simulink model "ASML_Simulate_KFilter"  (R2022a)
settings: Solver=FixedStepAuto  StartTime=0.0  StopTime=1  FixedStep=Ts  RelTol=1e-3
model workspace (MAT data in the model file):
  enab = 1
  eol = 6
  euvTarget = Simulink.Parameter
  euvTarget.Value = 4.4
  euvTarget.DataType = 'auto'
  euvTarget.Complexity = 'real'
  euvTarget.Dimensions = [1 1]
values from neighbouring files (symbols this model uses):
  euvTarget = 5    [modelParams.mat]
  HitDelayMode = 'zeroShot'    [modelParams.mat]    (also in variantParams.mat)
  SenseDelayMode = 'twoShot'    [modelParams.mat]    (also in variantParams.mat)
  Ts = 20e-6    (= 2e-05)    [computeDose1Burst.m]    (also in computeDose1Burst_filtered.m; modelParams.mat)
undefined symbols (not defined in the file or in its folder): Discrete, Time
libraries: ctrlSharedLib x1, simulink x1
settings Model: Creator=rjacques  LastModifiedBy=maxcr
settings SolverCC: AlgebraicLoopSolver=TrustRegion
settings DataIOCC: ExternalInput=extInput_SimulateEuvControl  DSMLogging=off  SaveTime=off  ReturnWorkspaceOutputs=off
settings OptimizationCC: EfficientMapNaN2IntZero=off
settings DebuggingCC: AlgebraicLoopMsg=none  UnconnectedInputMsg=warning  UnconnectedOutputMsg=warning  UnconnectedLineMsg=warning  SFMachineParentedDataDiag=warning  ArithmeticOperatorsInVariantConditions=warning
settings HardwareCC: TargetBitPerPointer=64  TargetBitPerSizeT=64  TargetBitPerPtrDiffT=64  TargetLongLongMode=on  TargetIntDivRoundTo=Zero  TargetEndianess=LittleEndian  TargetWordSize=64  TargetHWDeviceType=MATLAB Host  ProdEqTarget=off
settings SFSimCC: SimUseLocalCustomCode=off  CustomCodeUndefinedFunction=UseInterfaceOnly
settings RTWCC: SystemTargetFile=accel.tlc  TemplateMakefile=accel_default_tmf  RTWVerbose=off  DLArmComputeVersion=19.05
settings CodeAppCC: MaxIdLength=128
settings STFCustomTargetCC: ConcurrentExecutionCompliant=on  MATLABClassNameForMDSCustomization=Simulink.SoftwareTarget.TargetSpecificTriggerConfigurationBase  SystemTargetFile=accel.tlc

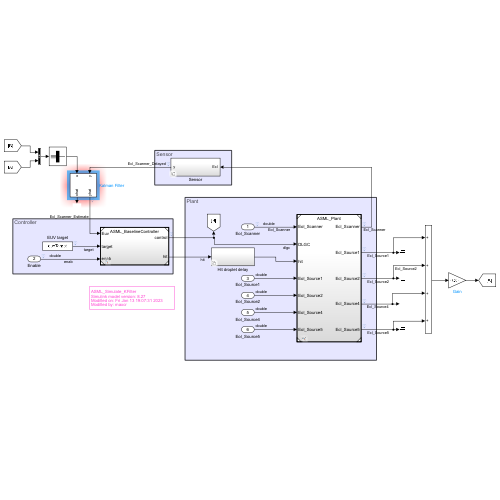
[thumbnail: Simulink's stored preview of the top-level diagram]
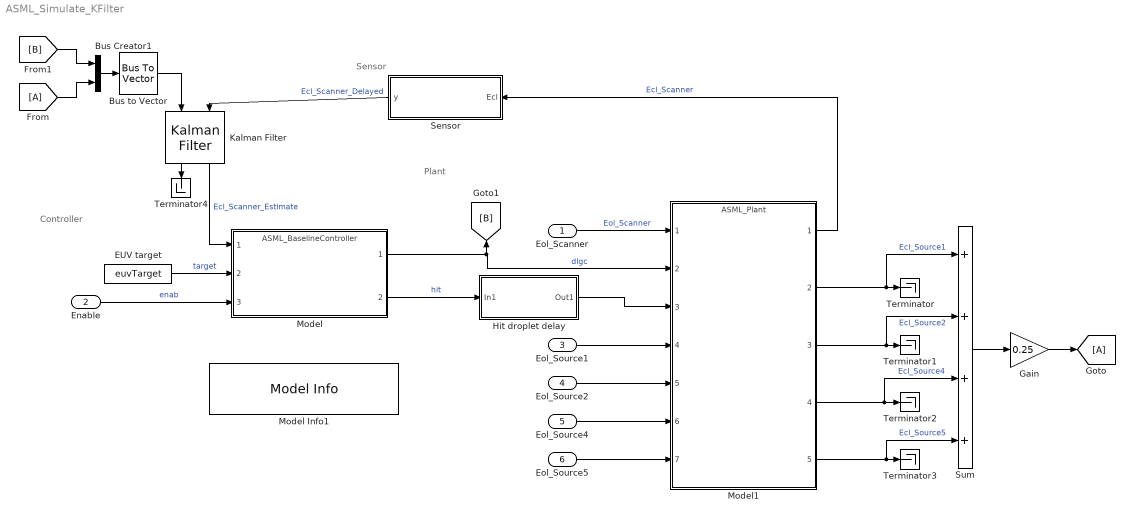
== system ASML_Simulate_KFilter ==
  note: Sensor
  note: Controller
  note: Plant
  Eol_Scanner : Inport  OutDataTypeStr=double  SampleTime=Ts
  Enable : Inport  Port=2  OutDataTypeStr=double  SampleTime=Ts
  Eol_Source1 : Inport  Port=3  OutDataTypeStr=double  SampleTime=Ts
  Eol_Source2 : Inport  Port=4  OutDataTypeStr=double  SampleTime=Ts
  Eol_Source4 : Inport  Port=5  OutDataTypeStr=double  SampleTime=Ts
  Eol_Source5 : Inport  Port=6  OutDataTypeStr=double  SampleTime=Ts
  Bus Creator1 : BusCreator  Inputs=2
  Bus to Vector : BusToVector
  EUV target : Constant  Value=euvTarget  OutDataTypeStr=double
  From : From
  Gain : Gain  Gain=0.25
  Goto : Goto
  Hit droplet delay : Subsystem  Variant=on
  Kalman Filter : ctrlSharedLib/Kalman Filter  TimeDomain=Discrete-Time  UseCurrentEstimator=off  ModelSource=LTI State-Space Variable  ModelSourceVariable=sys  A=0.95  B=1  C=1  D=0  NumberOfStates=1  NumberOfInputs=1  NumberOfOutputs=1  InitialEstimateSource=Dialog  X0=0  P0=10  UseK=off  UseGH=off  NumberOfProcessNoiseInputs=1  G=1  TimeInvariantG=on  H=0  TimeInvariantH=on  Q=0.05  TimeInvariantQ=on  R=1  TimeInvariantR=on  N=0  TimeInvariantN=on  AddInputPort=on  AddEnablePort=off  OutputEstimatedY=on  OutputP=off  Ts=-1
  Model : ModelReference  ModelNameDialog=ASML_BaselineController.slx  SimulationMode=Normal  ModelReferenceVersion=8.0
  Model Info1 : simulink/Model-Wide Utilities/Model Info  Frame=on  DisplayStringWithTags=|  HorizontalTextAlignment=Left  LeftAlignmentValue=0.02
      | %<ModelName>
      | Simulink model version: %<ModelVersion>
      | Modified on: %<LastModificationDate>
      | Modified by: %<ModifiedBy>
  Model1 : ModelReference  ModelNameDialog=ASML_Plant.slx  SimulationMode=Normal  ModelReferenceVersion=8.20
  Sensor : Subsystem  Variant=on  VariantControl=Variant1
  Sum : Sum  Inputs=++++
  Terminator{,1..4} (5 alike) : Terminator
  wires:
  Model/1 -> Model1/2, [B]  "dlgc"
  Eol_Scanner/1 -> Model1/1  "Eol_Scanner"
  EUV target/1 -> Model/2  "target"
  Model1/1 -> Sensor/1("Ecl ")  "Ecl_Scanner"
  Model/2 -> Hit droplet delay/1(In1)  "hit"
  Hit droplet delay/1(Out1) -> Model1/3
  Sensor/1(" y") -> Kalman Filter/2  "Ecl_Scanner_Delayed"
  Enable/1 -> Model/3  "enab"
  Eol_Source1/1 -> Model1/4
  Eol_Source2/1 -> Model1/5
  Eol_Source4/1 -> Model1/6
  Eol_Source5/1 -> Model1/7
  Model1/3 -> Sum/2, Terminator1/1  "Ecl_Source2"
  Model1/4 -> Sum/3, Terminator2/1  "Ecl_Source4"
  Model1/5 -> Sum/4, Terminator3/1  "Ecl_Source5"
  Model1/2 -> Sum/1, Terminator/1  "Ecl_Source1"
  Kalman Filter/2 -> Model/1  "Ecl_Scanner_Estimate"
  Bus Creator1/1 -> Bus to Vector/1
  Bus to Vector/1 -> Kalman Filter/1
  From/1 -> Bus Creator1/2
  [B] -> Bus Creator1/1
  Kalman Filter/1 -> Terminator4/1
  Sum/1 -> Gain/1
  Gain/1 -> Goto/1

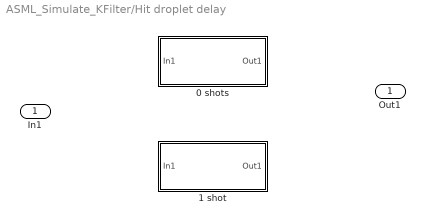
== system ASML_Simulate_KFilter/Hit droplet delay ==
  In1 : Inport
  0 shots : Subsystem  VariantControl=strcmp(HitDelayMode,'zeroShot')
  1 shot : Subsystem  VariantControl=strcmp(HitDelayMode,'oneShot')
  Out1 : Outport  VectorParamsAs1DForOutWhenUnconnected=off

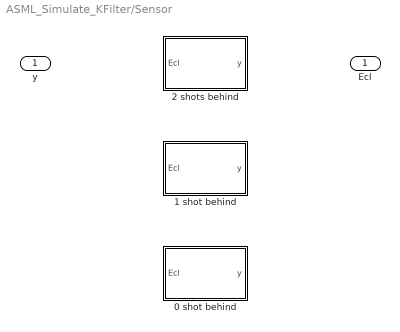
== system ASML_Simulate_KFilter/Sensor ==
  "Ecl " : Inport
  0 shot behind : Subsystem  VariantControl=strcmp(SenseDelayMode,'zeroShot')
  1 shot behind : Subsystem  VariantControl=strcmp(SenseDelayMode,'oneShot')
  2 shots behind : Subsystem  VariantControl=strcmp(SenseDelayMode,'twoShot')
  " y" : Outport  VectorParamsAs1DForOutWhenUnconnected=off

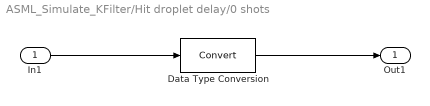
== system ASML_Simulate_KFilter/Hit droplet delay/0 shots ==
  In1 : Inport
  Data Type Conversion : DataTypeConversion  SaturateOnIntegerOverflow=off  RndMeth=Floor
  Out1 : Outport  VectorParamsAs1DForOutWhenUnconnected=off
  wires:
  In1/1 -> Data Type Conversion/1
  Data Type Conversion/1 -> Out1/1

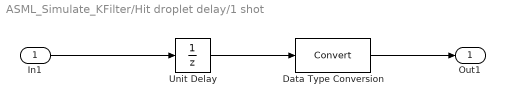
== system ASML_Simulate_KFilter/Hit droplet delay/1 shot ==
  In1 : Inport
  Data Type Conversion : DataTypeConversion  SaturateOnIntegerOverflow=off  RndMeth=Floor
  Unit Delay : UnitDelay  InitialCondition=1  SampleTime=-1  HasFrameUpgradeWarning=on
  Out1 : Outport  VectorParamsAs1DForOutWhenUnconnected=off
  wires:
  Unit Delay/1 -> Data Type Conversion/1
  In1/1 -> Unit Delay/1
  Data Type Conversion/1 -> Out1/1

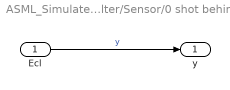
== system ASML_Simulate_KFilter/Sensor/0 shot behind ==
  Ecl : Inport
  y : Outport  VectorParamsAs1DForOutWhenUnconnected=off
  wires:
  Ecl/1 -> y/1  "y"

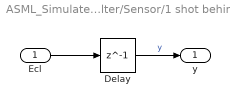
== system ASML_Simulate_KFilter/Sensor/1 shot behind ==
  Ecl : Inport
  Delay : Delay  DelayLength=1  InitialCondition=5
  y : Outport  VectorParamsAs1DForOutWhenUnconnected=off
  wires:
  Ecl/1 -> Delay/1
  Delay/1 -> y/1  "y"

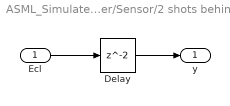
== system ASML_Simulate_KFilter/Sensor/2 shots behind ==
  Ecl : Inport
  Delay : Delay  InitialCondition=5
  y : Outport  VectorParamsAs1DForOutWhenUnconnected=off
  wires:
  Delay/1 -> y/1
  Ecl/1 -> Delay/1
